simulink model "ASM2d_Influentmodel"  (Simulink 7.0)
settings: Solver=ode45  StartTime=0.0  StopTime=728.0  RelTol=1e-6
values from neighbouring files (symbols this model uses):
  aHpercent = 75    [ASM2d_Influent_init.m]    (also in ASM3_Influent_init.m)
  CODpart_gperPEperd = 115.08    [ASM2d_Influent_init.m]    (also in ASM3_Influent_init.m)
  CODpart_HH_max = 20*CODpart_gperPEperd*PE    (= 184128)    [ASM2d_Influent_init.m]    (also in ASM3_Influent_init.m)
  CODpart_HH_min = 0.1    [ASM2d_Influent_init.m]    (also in ASM3_Influent_init.m)
  CODpart_HH_ns = 35000    [ASM2d_Influent_init.m]    (also in ASM3_Influent_init.m)
  CODpart_HH_nv = factor1*CODpart_gperPEperd*PE    (= 18412.8)    [ASM2d_Influent_init.m]    (also in ASM3_Influent_init.m)
  CODpart_HH_st = 1/24    (= 0.0416666666667)    [ASM2d_Influent_init.m]    (also in ASM3_Influent_init.m)
  CODpart_Ind_kgperd = 2301.80    (= 2301.8)    [ASM2d_Influent_init.m]    (also in ASM3_Influent_init.m)
  CODpart_Ind_max = 20*CODpart_Ind_kgperd    (= 46036)    [ASM2d_Influent_init.m]    (also in ASM3_Influent_init.m)
  CODpart_Ind_min = 0.1    [ASM2d_Influent_init.m]    (also in ASM3_Influent_init.m)
  CODpart_Ind_ns = 21000    [ASM2d_Influent_init.m]    (also in ASM3_Influent_init.m)
  CODpart_Ind_nv = factor2*CODpart_Ind_kgperd    (= 4603.6)    [ASM2d_Influent_init.m]    (also in ASM3_Influent_init.m)
  CODpart_Ind_st = 1/24    (= 0.0416666666667)    [ASM2d_Influent_init.m]    (also in ASM3_Influent_init.m)
  CODsol_gperPEperd = 19.31    [ASM2d_Influent_init.m]    (also in ASM3_Influent_init.m)
  CODsol_HH_max = 20*CODsol_gperPEperd*PE    (= 30896)    [ASM2d_Influent_init.m]    (also in ASM3_Influent_init.m)
  CODsol_HH_min = 0.1    [ASM2d_Influent_init.m]    (also in ASM3_Influent_init.m)
  CODsol_HH_ns = 25000    [ASM2d_Influent_init.m]    (also in ASM3_Influent_init.m)
  CODsol_HH_nv = factor1*2*CODsol_gperPEperd*PE    (= 6179.2)    [ASM2d_Influent_init.m]    (also in ASM3_Influent_init.m)
  CODsol_HH_st = 1/24    (= 0.0416666666667)    [ASM2d_Influent_init.m]    (also in ASM3_Influent_init.m)
  CODsol_Ind_kgperd = 386.24    [ASM2d_Influent_init.m]    (also in ASM3_Influent_init.m)
  CODsol_Ind_max = 20*CODsol_Ind_kgperd    (= 7724.8)    [ASM2d_Influent_init.m]    (also in ASM3_Influent_init.m)
  CODsol_Ind_min = 0.1    [ASM2d_Influent_init.m]    (also in ASM3_Influent_init.m)
  CODsol_Ind_ns = 11000    [ASM2d_Influent_init.m]    (also in ASM3_Influent_init.m)
  CODsol_Ind_nv = factor2*CODsol_Ind_kgperd    (= 772.48)    [ASM2d_Influent_init.m]    (also in ASM3_Influent_init.m)
  CODsol_Ind_st = 1/24    (= 0.0416666666667)    [ASM2d_Influent_init.m]    (also in ASM3_Influent_init.m)
  FFfraction = 0.25    [ASM2d_Influent_init.m]    (also in ASM3_Influent_init.m)
  HHnoiseswitch = 1    [ASM2d_Influent_init.m]    (also in ASM3_Influent_init.m)
  HHpolnoiseswitch = 1    [ASM2d_Influent_init.m]    (also in ASM3_Influent_init.m)
  HHpopswitch = 100    [ASM2d_Influent_init.m]    (also in ASM3_Influent_init.m)
  Indnoiseswitch = 1    [ASM2d_Influent_init.m]    (also in ASM3_Influent_init.m)
  Indpolnoiseswitch = 1    [ASM2d_Influent_init.m]    (also in ASM3_Influent_init.m)
  Indpopswitch = 100    [ASM2d_Influent_init.m]    (also in ASM3_Influent_init.m)
  InfAmp = 1200    [ASM2d_Influent_init.m]    (also in ASM3_Influent_init.m)
  InfBias = 7100    [ASM2d_Influent_init.m]    (also in ASM3_Influent_init.m)
  Infcst = 7100    [ASM2d_Influent_init.m]    (also in ASM3_Influent_init.m)
  InfFreq = 2*pi/364    (= 0.0172614980966)    [ASM2d_Influent_init.m]    (also in ASM3_Influent_init.m)
  InfPhase = -pi*15/24    (= -1.96349540849)    [ASM2d_Influent_init.m]    (also in ASM3_Influent_init.m)
  iSS_XB = 0.90    (= 0.9)    [ASM2d_Influent_init.m]
  iSS_XI = 0.75    [ASM2d_Influent_init.m]
  iSS_XMe = 1.00    (= 1)    [ASM2d_Influent_init.m]
  iSS_XPHA = 0.60    (= 0.6)    [ASM2d_Influent_init.m]
  iSS_XPP = 3.23    [ASM2d_Influent_init.m]
  iSS_XS = 0.75    [ASM2d_Influent_init.m]
  LLrain = 3.5    [ASM2d_Influent_init.m]    (also in ASM3_Influent_init.m)
  PE = 80    [ASM2d_Influent_init.m]    (also in ASM3_Influent_init.m)
  PO4_gperPEperd = (6.89*0.85)/4    (= 1.464125)    [ASM2d_Influent_init.m]
  PO4_HH_max = 20*PO4_gperPEperd*PE    (= 2342.6)    [ASM2d_Influent_init.m]
  PO4_HH_min = 0.1    [ASM2d_Influent_init.m]
  PO4_HH_ns = 55000    [ASM2d_Influent_init.m]
  PO4_HH_nv = factor1*2*PO4_gperPEperd*PE    (= 468.52)    [ASM2d_Influent_init.m]
  PO4_HH_st = 1/24    (= 0.0416666666667)    [ASM2d_Influent_init.m]
  PO4_Ind_kgperd = (61.25*0.85)/4    (= 13.015625)    [ASM2d_Influent_init.m]
  PO4_Ind_max = 20*PO4_Ind_kgperd    (= 260.3125)    [ASM2d_Influent_init.m]
  PO4_Ind_min = 0.1    [ASM2d_Influent_init.m]
  PO4_Ind_ns = 41000    [ASM2d_Influent_init.m]
  PO4_Ind_nv = factor2*PO4_Ind_kgperd    (= 26.03125)    [ASM2d_Influent_init.m]
  PO4_Ind_st = 1/24    (= 0.0416666666667)    [ASM2d_Influent_init.m]
  polnoiseswitch = 1    [ASM2d_Influent_init.m]    (also in ASM3_Influent_init.m)
  Q_HH_ns = 3857    [ASM2d_Influent_init.m]    (also in ASM3_Influent_init.m)
  Q_HH_nv = 4000    [ASM2d_Influent_init.m]    (also in ASM3_Influent_init.m)
  Q_HH_st = 1/24    (= 0.0416666666667)    [ASM2d_Influent_init.m]    (also in ASM3_Influent_init.m)
  Q_Ind_ns = 2000    [ASM2d_Influent_init.m]    (also in ASM3_Influent_init.m)
  Q_Ind_nv = 15000    [ASM2d_Influent_init.m]    (also in ASM3_Influent_init.m)
  Q_Ind_st = 1/24    (= 0.0416666666667)    [ASM2d_Influent_init.m]    (also in ASM3_Influent_init.m)
  Q_SCI_ns = 1000    [ASM2d_Influent_init.m]    (also in ASM3_Influent_init.m)
  Q_SCI_nv = 0.1*InfBias    (= 710)    [ASM2d_Influent_init.m]    (also in ASM3_Influent_init.m)
  Q_SCI_st = 1    [ASM2d_Influent_init.m]    (also in ASM3_Influent_init.m)
  QHHsatmax = QperPE*50    (= 7500)    [ASM2d_Influent_init.m]    (also in ASM3_Influent_init.m)
  QHHsatmin = 0.001    [ASM2d_Influent_init.m]    (also in ASM3_Influent_init.m)
  QInd_weekday = 2500    [ASM2d_Influent_init.m]    (also in ASM3_Influent_init.m)
  QIndsatmax = QInd_weekday*10    (= 25000)    [ASM2d_Influent_init.m]    (also in ASM3_Influent_init.m)
  QIndsatmin = 0.001    [ASM2d_Influent_init.m]    (also in ASM3_Influent_init.m)
  Qpermm = 1500    [ASM2d_Influent_init.m]    (also in ASM3_Influent_init.m)
  QperPE = 150    [ASM2d_Influent_init.m]    (also in ASM3_Influent_init.m)
  QSCIsatmax = 2*(InfBias+InfAmp)    (= 16600)    [ASM2d_Influent_init.m]    (also in ASM3_Influent_init.m)
  QSCIsatmin = 0.0    (= 0)    [ASM2d_Influent_init.m]    (also in ASM3_Influent_init.m)
  rain_nm = 1    [ASM2d_Influent_init.m]    (also in ASM3_Influent_init.m)
  rain_ns = 3000    [ASM2d_Influent_init.m]    (also in ASM3_Influent_init.m)
  rain_nv = 400    [ASM2d_Influent_init.m]    (also in ASM3_Influent_init.m)
  rain_st = 1/24    (= 0.0416666666667)    [ASM2d_Influent_init.m]    (also in ASM3_Influent_init.m)
  rainmax = 1000    [ASM2d_Influent_init.m]    (also in ASM3_Influent_init.m)
  rainmin = 0    [ASM2d_Influent_init.m]    (also in ASM3_Influent_init.m)
  rainpopswitch = 100    [ASM2d_Influent_init.m]    (also in ASM3_Influent_init.m)
  SA_max = 100*Sa_in    (= 2780)    [ASM2d_Influent_init.m]
  SA_min = 0.1    [ASM2d_Influent_init.m]
  SA_ns = 03122    (= 3122)    [ASM2d_Influent_init.m]
  SA_nv = factor3*(Sa_in)    (= 55.6)    [ASM2d_Influent_init.m]
  SA_st = 1/24    (= 0.0416666666667)    [ASM2d_Influent_init.m]
  SCInoiseswitch = 0    [ASM2d_Influent_init.m]    (also in ASM3_Influent_init.m)
  SCIpopswitch = 100    [ASM2d_Influent_init.m]    (also in ASM3_Influent_init.m)
  SF_max = 100*Sf_in    (= 4170)    [ASM2d_Influent_init.m]
  SF_min = 0.1    [ASM2d_Influent_init.m]
  SF_ns = 23122    [ASM2d_Influent_init.m]
  SF_nv = factor3*(Sf_in)    (= 83.4)    [ASM2d_Influent_init.m]
  SF_st = 1/24    (= 0.0416666666667)    [ASM2d_Influent_init.m]
  SI_max = 100*Si_in    (= 3000)    [ASM2d_Influent_init.m]    (also in ASM3_Influent_init.m)
  SI_min = 0.1    [ASM2d_Influent_init.m]    (also in ASM3_Influent_init.m)
  SI_ns = 13122    [ASM2d_Influent_init.m]    (also in ASM3_Influent_init.m)
  SI_nv = factor3*(Si_in)    (= 60)    [ASM2d_Influent_init.m]    (also in ASM3_Influent_init.m)
  SI_st = 1/24    (= 0.0416666666667)    [ASM2d_Influent_init.m]    (also in ASM3_Influent_init.m)
  SNH_gperPEperd = 6.89*0.85    (= 5.8565)    [ASM2d_Influent_init.m]    (also in ASM3_Influent_init.m)
  SNH_HH_max = 20*SNH_gperPEperd*PE    (= 9370.4)    [ASM2d_Influent_init.m]    (also in ASM3_Influent_init.m)
  SNH_HH_min = 0.1    [ASM2d_Influent_init.m]    (also in ASM3_Influent_init.m)
  SNH_HH_ns = 45000    [ASM2d_Influent_init.m]    (also in ASM3_Influent_init.m)
  SNH_HH_nv = factor1*2*SNH_gperPEperd*PE    (= 1874.08)    [ASM2d_Influent_init.m]    (also in ASM3_Influent_init.m)
  SNH_HH_st = 1/24    (= 0.0416666666667)    [ASM2d_Influent_init.m]    (also in ASM3_Influent_init.m)
  SNH_Ind_kgperd = 61.25*0.85    (= 52.0625)    [ASM2d_Influent_init.m]    (also in ASM3_Influent_init.m)
  SNH_Ind_max = 20*SNH_Ind_kgperd    (= 1041.25)    [ASM2d_Influent_init.m]    (also in ASM3_Influent_init.m)
  SNH_Ind_min = 0.1    [ASM2d_Influent_init.m]    (also in ASM3_Influent_init.m)
  SNH_Ind_ns = 31000    [ASM2d_Influent_init.m]    (also in ASM3_Influent_init.m)
  SNH_Ind_nv = factor2*SNH_Ind_kgperd    (= 104.125)    [ASM2d_Influent_init.m]    (also in ASM3_Influent_init.m)
  SNH_Ind_st = 1/24    (= 0.0416666666667)    [ASM2d_Influent_init.m]    (also in ASM3_Influent_init.m)
  SNH_max = 100*Snh_in    (= 3156)    [ASM2d_Influent_init.m]    (also in ASM3_Influent_init.m)
  SNH_min = 0.1    [ASM2d_Influent_init.m]    (also in ASM3_Influent_init.m)
  SNH_ns = 63122    [ASM2d_Influent_init.m]    (also in ASM3_Influent_init.m)
  SNH_nv = factor3*(Snh_in)    (= 63.12)    [ASM2d_Influent_init.m]    (also in ASM3_Influent_init.m)
  SNH_st = 1/24    (= 0.0416666666667)    [ASM2d_Influent_init.m]    (also in ASM3_Influent_init.m)
  SPO4_ns = 73122    [ASM2d_Influent_init.m]
  SPO4_nv = factor3*(Spo4_in)    (= 18.02)    [ASM2d_Influent_init.m]
  SPO4_st = 1/24    (= 0.0416666666667)    [ASM2d_Influent_init.m]
  ... (+24 more)
libraries: simulink x5
(part 1 of 2)
Description:
  | BSM2 influent model, version 15 March 2005
settings Model: Creator=Krist V. Gernaey  LastModifiedBy=xavier  ExtModeAutoUpdateStatusClock=off
settings DataIOCC: LimitDataPoints=off  SignalLoggingName=sigsOut  OutputOption=SpecifiedOutputTimes  OutputTimes=[119:1.0/96.0:728.0]
settings DebuggingCC: SaveWithParameterizedLinksMsg=none  SignalResolutionControl=TryResolveAllWithWarning  SolverPrmCheckMsg=none  MultiTaskDSMMsg=warning  MultiTaskCondExecSysMsg=none  StrictBusMsg=None
settings HardwareCC: TargetEndianess=LittleEndian  TargetHWDeviceType=MATLAB Host  ProdEqTarget=off
settings RTWCC: IncludeERTFirstTime=on

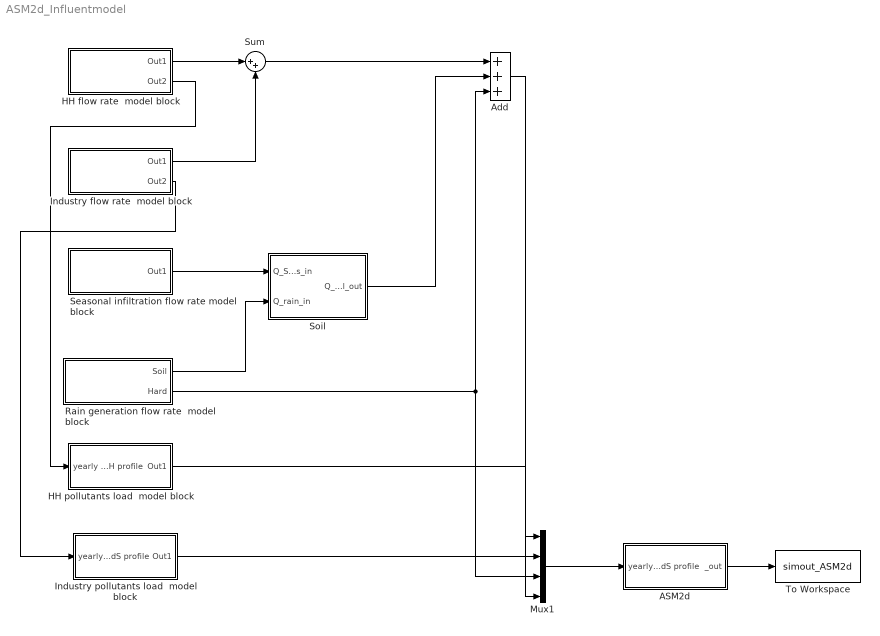
== system ASM2d_Influentmodel ==
  ASM2d : Subsystem
  Add : Sum  Inputs=+++  OutDataType=sfix(16)  OutScaling=2^-10
  HH flow rate  model block : Subsystem
  "HH pollutants load  model block " : Subsystem
  Industry flow rate  model block : Subsystem
  "Industry pollutants load  model block " : Subsystem
  Mux1 : Mux
  Rain generation flow rate  model block : Subsystem
  Seasonal infiltration flow rate model block : Subsystem
  Soil : Subsystem
  Sum : Sum  Inputs=|++  OutDataType=sfix(16)  OutScaling=2^0  SaturateOnIntegerOverflow=on
  To Workspace : ToWorkspace  VariableName=simout_ASM2d  SampleTime=-1  SaveFormat=Array
  wires:
  Add/1 -> Mux1/4
  Rain generation flow rate  model block/2(Hard) -> Mux1/3, Add/3
  Soil/1(Q_Soil_out) -> Add/2
  Sum/1 -> Add/1
  HH flow rate  model block/1(Out1) -> Sum/1
  Rain generation flow rate  model block/1(Soil) -> Soil/2(Q_rain_in)
  Seasonal infiltration flow rate model block/1(Out1) -> Soil/1(Q_Seas_in)
  Industry flow rate  model block/1(Out1) -> Sum/2
  HH flow rate  model block/2(Out2) -> "HH pollutants load  model block "/1(yearly HH profile)
  Industry flow rate  model block/2(Out2) -> "Industry pollutants load  model block "/1(yearly_indS profile)
  "HH pollutants load  model block "/1(Out1) -> Mux1/1
  "Industry pollutants load  model block "/1(Out1) -> Mux1/2
  Mux1/1 -> ASM2d/1(yearly_indS profile)
  ASM2d/1(_out) -> To Workspace/1

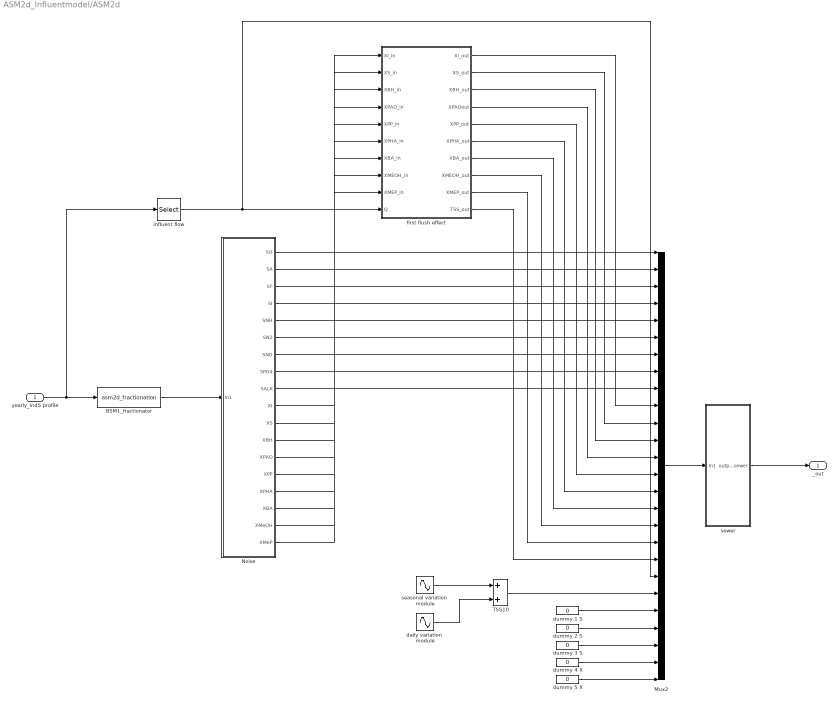
== system ASM2d_Influentmodel/ASM2d ==
  yearly_indS profile : Inport  OutDataType=sfix(16)  OutScaling=2^0
  BSM1_fractionator : S-Function  FunctionName=asm2d_fractionation  Parameters=ASM2d_PARS, ASM2d_FRACTIONS
  Mux2 : Mux  Inputs=26
  Noise : Subsystem
  TSS10 : Sum  OutDataType=sfix(16)  OutScaling=2^-10
  daily variation  module : Sin  Amplitude=TdAmp  Bias=TdBias  Frequency=TdFreq  Phase=TdPhase  SampleTime=0
  dummy 1 S : Constant  Value=0  OutDataType=sfix(16)  OutScaling=2^0
  dummy 2 S : Constant  Value=0  OutDataType=sfix(16)  OutScaling=2^0
  dummy 3 S : Constant  Value=0  OutDataType=sfix(16)  OutScaling=2^0
  dummy 4 X : Constant  Value=0  OutDataType=sfix(16)  OutScaling=2^0
  dummy 5 X : Constant  Value=0  OutDataType=sfix(16)  OutScaling=2^0
  first flush effect : Subsystem
  influent flow : Selector  InputPortWidth=12  IndexOptions=Index vector (dialog)  Indices=[12]  OutputSizes=1
  seasonal variation  module : Sin  Amplitude=TAmp  Bias=TBias  Frequency=TFreq  Phase=TPhase  SampleTime=0
  sewer : Subsystem
  _out : Outport  OutDataType=sfix(16)  OutScaling=2^0
  wires:
  yearly_indS profile/1 -> BSM1_fractionator/1, influent flow/1
  Noise/10(XI) -> first flush effect/1(XI_in)
  Noise/11(XS) -> first flush effect/2(XS_in)
  Noise/12(XBH) -> first flush effect/3(XBH_in)
  Noise/13(XPAO) -> first flush effect/4(XPAO_in)
  Noise/14(XPP) -> first flush effect/5(XPP_in)
  Noise/15(XPHA) -> first flush effect/6(XPHA_in)
  Noise/16(XBA) -> first flush effect/7(XBA_in)
  Noise/17(XMeOH) -> first flush effect/8(XMEOH_in)
  Noise/18(XMeP) -> first flush effect/9(XMEP_in)
  BSM1_fractionator/1 -> Noise/1(In1)
  influent flow/1 -> first flush effect/10(Q), Mux2/20
  Noise/1(SO) -> Mux2/1
  Noise/2(SA) -> Mux2/2
  Noise/3(SF) -> Mux2/3
  Noise/4(SI) -> Mux2/4
  Noise/5(SNH) -> Mux2/5
  Noise/6(SN2) -> Mux2/6
  Noise/7(SNO) -> Mux2/7
  Noise/8(SPO4) -> Mux2/8
  Noise/9(SALK) -> Mux2/9
  first flush effect/1(XI_out) -> Mux2/10
  first flush effect/2(XS_out) -> Mux2/11
  first flush effect/3(XBH_out) -> Mux2/12
  first flush effect/4(XPAOout) -> Mux2/13
  first flush effect/5(XPP_out) -> Mux2/14
  first flush effect/6(XPHA_out) -> Mux2/15
  first flush effect/7(XBA_out) -> Mux2/16
  first flush effect/8(XMEOH_out) -> Mux2/17
  first flush effect/9(XMEP_out) -> Mux2/18
  first flush effect/10(TSS_out) -> Mux2/19
  dummy 5 X/1 -> Mux2/26
  dummy 4 X/1 -> Mux2/25
  dummy 3 S/1 -> Mux2/24
  dummy 2 S/1 -> Mux2/23
  dummy 1 S/1 -> Mux2/22
  Mux2/1 -> sewer/1(In1)
  sewer/1(output sewer) -> _out/1
  TSS10/1 -> Mux2/21
  seasonal variation  module/1 -> TSS10/1
  daily variation  module/1 -> TSS10/2

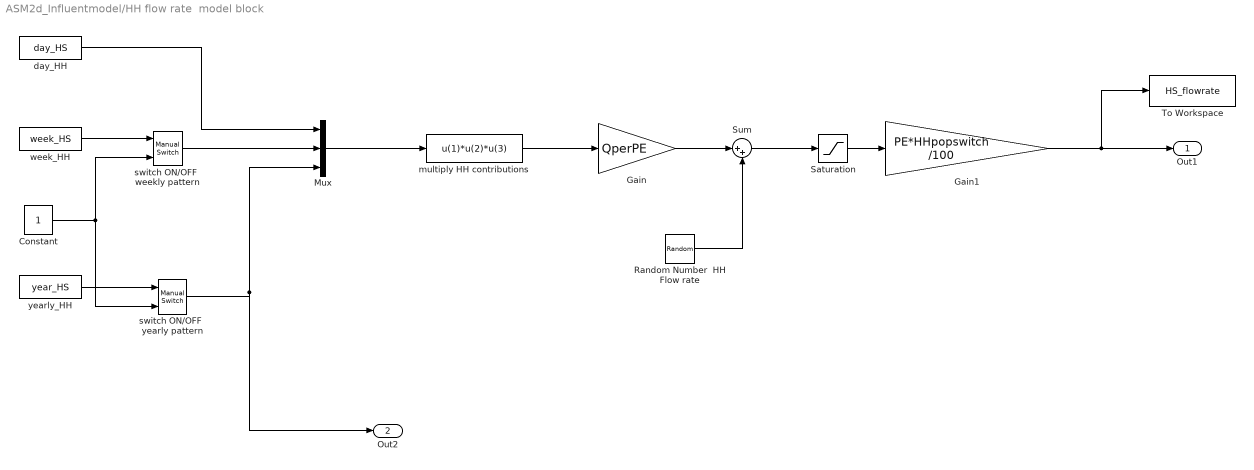
== system ASM2d_Influentmodel/HH flow rate  model block ==
  Constant : Constant  OutDataType=sfix(16)  OutScaling=2^0
  Gain : Gain  Gain=QperPE  ParameterDataType=sfix(16)  ParameterScaling=2^0  OutDataType=sfix(16)  OutScaling=2^0
  Gain1 : Gain  Gain=PE*HHpopswitch /100  ParameterDataType=sfix(16)  ParameterScaling=2^0  OutDataType=sfix(16)  OutScaling=2^0
  Mux : Mux  Inputs=3
  Random Number  HH Flow rate : RandomNumber  Variance=Q_HH_nv*HHnoiseswitch  Seed=Q_HH_ns  SampleTime=Q_HH_st
  Saturation : Saturate  UpperLimit=QHHsatmax  LowerLimit=QHHsatmin  OutDataType=sfix(16)  OutScaling=2^0
  Sum : Sum  Inputs=|++  OutDataType=sfix(16)  OutScaling=2^0
  To Workspace : ToWorkspace  VariableName=HS_flowrate  SampleTime=-1  SaveFormat=Array
  day_HH : FromWorkspace  VariableName=day_HS  SampleTime=1/24  Interpolate=off  OutputAfterFinalValue=Cyclic repetition
  multiply HH contributions : Fcn  Expr=u(1)*u(2)*u(3)
  switch ON/OFF  weekly pattern : simulink/Signal Routing/Manual Switch  SystemSampleTime=-1  sw=1  action=0  varsize=off
  switch ON/OFF  yearly pattern : simulink/Signal Routing/Manual Switch  SystemSampleTime=-1  sw=1  action=0  varsize=off
  week_HH : FromWorkspace  VariableName=week_HS  SampleTime=1  Interpolate=off  OutputAfterFinalValue=Cyclic repetition
  yearly_HH : FromWorkspace  VariableName=year_HS  SampleTime=1  Interpolate=off  OutputAfterFinalValue=Cyclic repetition
  Out1 : Outport  OutDataType=sfix(16)  OutScaling=2^0
  Out2 : Outport  Port=2  OutDataType=sfix(16)  OutScaling=2^0
  wires:
  multiply HH contributions/1 -> Gain/1
  Gain/1 -> Sum/1
  Sum/1 -> Saturation/1
  Saturation/1 -> Gain1/1
  Gain1/1 -> Out1/1, To Workspace/1
  Random Number  HH Flow rate/1 -> Sum/2
  week_HH/1 -> switch ON/OFF  weekly pattern/1
  yearly_HH/1 -> switch ON/OFF  yearly pattern/1
  day_HH/1 -> Mux/1
  switch ON/OFF  weekly pattern/1 -> Mux/2
  switch ON/OFF  yearly pattern/1 -> Mux/3, Out2/1
  Constant/1 -> switch ON/OFF  weekly pattern/2, switch ON/OFF  yearly pattern/2
  Mux/1 -> multiply HH contributions/1

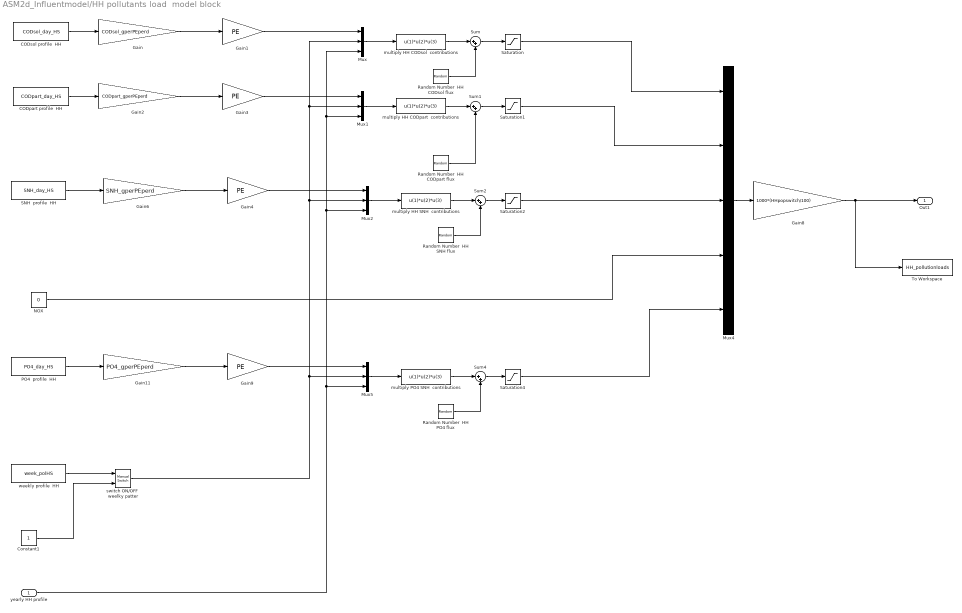
== system ASM2d_Influentmodel/HH pollutants load  model block  ==
  yearly HH profile : Inport  OutDataType=sfix(16)  OutScaling=2^0
  CODpart profile  HH : FromWorkspace  VariableName=CODpart_day_HS  SampleTime=1/24  Interpolate=off  OutputAfterFinalValue=Cyclic repetition
  CODsol profile  HH : FromWorkspace  VariableName=CODsol_day_HS  SampleTime=1/24  Interpolate=off  OutputAfterFinalValue=Cyclic repetition
  Constant1 : Constant  OutDataType=sfix(16)  OutScaling=2^0
  Gain : Gain  Gain=CODsol_gperPEperd  ParameterDataType=sfix(16)  ParameterScaling=2^0  OutDataType=sfix(16)  OutScaling=2^0
  Gain{1,3..4,9} (4 alike) : Gain  Gain=PE  ParameterDataType=sfix(16)  ParameterScaling=2^0  OutDataType=sfix(16)  OutScaling=2^0
  Gain11 : Gain  Gain=PO4_gperPEperd  ParameterDataType=sfix(16)  ParameterScaling=2^0  OutDataType=sfix(16)  OutScaling=2^0
  Gain2 : Gain  Gain=CODpart_gperPEperd  ParameterDataType=sfix(16)  ParameterScaling=2^0  OutDataType=sfix(16)  OutScaling=2^0
  Gain6 : Gain  Gain=SNH_gperPEperd  ParameterDataType=sfix(16)  ParameterScaling=2^0  OutDataType=sfix(16)  OutScaling=2^0
  Gain8 : Gain  Gain=1000*(HHpopswitch/100)  ParameterDataType=sfix(16)  ParameterScaling=2^0  OutDataType=sfix(16)  OutScaling=2^0
  Mux{,1..2,5} (4 alike) : Mux  Inputs=3
  Mux4 : Mux  Inputs=5
  NOX : Constant  Value=0  OutDataType=sfix(16)  OutScaling=2^0
  PO4  profile  HH : FromWorkspace  VariableName=PO4_day_HS  SampleTime=1/24  Interpolate=off  OutputAfterFinalValue=Cyclic repetition
  Random Number  HH CODpart flux : RandomNumber  Variance=CODpart_HH_nv*HHpolnoiseswitch  Seed=CODpart_HH_ns  SampleTime=CODpart_HH_st
  Random Number  HH CODsol flux : RandomNumber  Variance=CODsol_HH_nv*HHpolnoiseswitch  Seed=CODsol_HH_ns  SampleTime=CODsol_HH_st
  Random Number  HH PO4 flux : RandomNumber  Variance=PO4_HH_nv*HHpolnoiseswitch  Seed=PO4_HH_ns  SampleTime=PO4_HH_st
  Random Number  HH SNH flux : RandomNumber  Variance=SNH_HH_nv*HHpolnoiseswitch  Seed=SNH_HH_ns  SampleTime=SNH_HH_st
  SNH  profile  HH : FromWorkspace  VariableName=SNH_day_HS  SampleTime=1/24  Interpolate=off  OutputAfterFinalValue=Cyclic repetition
  Saturation : Saturate  UpperLimit=CODsol_HH_max  LowerLimit=CODsol_HH_min  OutDataType=sfix(16)  OutScaling=2^0
  Saturation1 : Saturate  UpperLimit=CODpart_HH_max  LowerLimit=CODpart_HH_min  OutDataType=sfix(16)  OutScaling=2^0
  Saturation2 : Saturate  UpperLimit=SNH_HH_max  LowerLimit=SNH_HH_min  OutDataType=sfix(16)  OutScaling=2^0
  Saturation4 : Saturate  UpperLimit=PO4_HH_max  LowerLimit=PO4_HH_min  OutDataType=sfix(16)  OutScaling=2^0
  Sum{,1..2,4} (4 alike) : Sum  Inputs=|++  OutDataType=sfix(16)  OutScaling=2^0
  To Workspace : ToWorkspace  VariableName=HH_pollutionloads  SampleTime=-1  SaveFormat=Array
  multiply HH CODpart  contributions : Fcn  Expr=u(1)*u(2)*u(3)
  multiply HH CODsol  contributions : Fcn  Expr=u(1)*u(2)*u(3)
  multiply HH SNH  contributions : Fcn  Expr=u(1)*u(2)*u(3)
  multiply PO4 SNH  contributions : Fcn  Expr=u(1)*u(2)*u(3)
  switch ON/OFF  weelky patter : simulink/Signal Routing/Manual Switch  SystemSampleTime=-1  sw=1  action=0  varsize=off
  weekly profile  HH : FromWorkspace  VariableName=week_polHS  SampleTime=1  Interpolate=off  OutputAfterFinalValue=Cyclic repetition
  Out1 : Outport  OutDataType=sfix(16)  OutScaling=2^0
  wires:
  Random Number  HH CODsol flux/1 -> Sum/2
  CODsol profile  HH/1 -> Gain/1
  Gain/1 -> Gain1/1
  Mux/1 -> multiply HH CODsol  contributions/1
  multiply HH CODsol  contributions/1 -> Sum/1
  Sum/1 -> Saturation/1
  Gain1/1 -> Mux/1
  Random Number  HH CODpart flux/1 -> Sum1/2
  CODpart profile  HH/1 -> Gain2/1
  Gain2/1 -> Gain3/1
  Mux1/1 -> multiply HH CODpart  contributions/1
  multiply HH CODpart  contributions/1 -> Sum1/1
  Sum1/1 -> Saturation1/1
  Gain3/1 -> Mux1/1
  Random Number  HH SNH flux/1 -> Sum2/2
  SNH  profile  HH/1 -> Gain6/1
  Gain6/1 -> Gain4/1
  Mux2/1 -> multiply HH SNH  contributions/1
  multiply HH SNH  contributions/1 -> Sum2/1
  Sum2/1 -> Saturation2/1
  Gain4/1 -> Mux2/1
  Mux4/1 -> Gain8/1
  Constant1/1 -> switch ON/OFF  weelky patter/2
  weekly profile  HH/1 -> switch ON/OFF  weelky patter/1
  Random Number  HH PO4 flux/1 -> Sum4/2
  PO4  profile  HH/1 -> Gain11/1
  Gain11/1 -> Gain9/1
  Mux5/1 -> multiply PO4 SNH  contributions/1
  multiply PO4 SNH  contributions/1 -> Sum4/1
  Sum4/1 -> Saturation4/1
  Gain9/1 -> Mux5/1
  Saturation/1 -> Mux4/1
  Saturation1/1 -> Mux4/2
  Saturation2/1 -> Mux4/3
  Saturation4/1 -> Mux4/5
  switch ON/OFF  weelky patter/1 -> Mux5/2, Mux2/2, Mux/2, Mux1/2
  yearly HH profile/1 -> Mux5/3, Mux2/3, Mux/3, Mux1/3
  Gain8/1 -> Out1/1, To Workspace/1
  NOX/1 -> Mux4/4

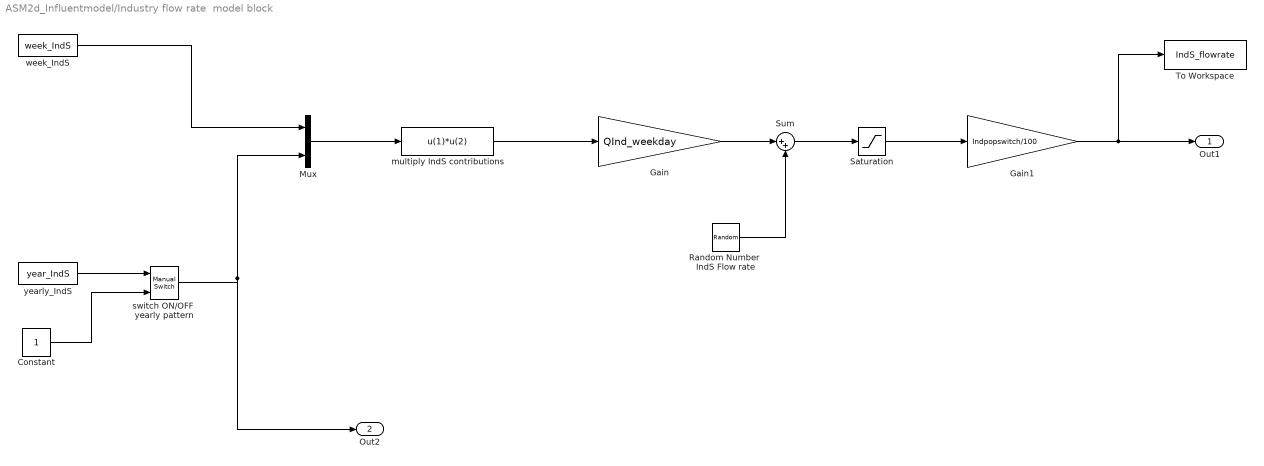
== system ASM2d_Influentmodel/Industry flow rate  model block ==
  Constant : Constant  OutDataType=sfix(16)  OutScaling=2^0
  Gain : Gain  Gain=QInd_weekday  ParameterDataType=sfix(16)  ParameterScaling=2^0  OutDataType=sfix(16)  OutScaling=2^0
  Gain1 : Gain  Gain=Indpopswitch/100  ParameterDataType=sfix(16)  ParameterScaling=2^0  OutDataType=sfix(16)  OutScaling=2^0
  Mux : Mux  Inputs=2
  Random Number  IndS Flow rate : RandomNumber  Variance=Q_Ind_nv*Indnoiseswitch  Seed=Q_Ind_ns  SampleTime=Q_Ind_st
  Saturation : Saturate  UpperLimit=QIndsatmax  LowerLimit=QIndsatmin  OutDataType=sfix(16)  OutScaling=2^0
  Sum : Sum  Inputs=|++  OutDataType=sfix(16)  OutScaling=2^0
  To Workspace : ToWorkspace  VariableName=IndS_flowrate  SampleTime=-1  SaveFormat=Array
  multiply IndS contributions : Fcn  Expr=u(1)*u(2)
  switch ON/OFF  yearly pattern : simulink/Signal Routing/Manual Switch  SystemSampleTime=-1  sw=1  action=0  varsize=off
  week_IndS : FromWorkspace  VariableName=week_IndS  SampleTime=1/6  Interpolate=off  OutputAfterFinalValue=Cyclic repetition
  yearly_IndS : FromWorkspace  VariableName=year_IndS  SampleTime=1  Interpolate=off  OutputAfterFinalValue=Cyclic repetition
  Out1 : Outport  OutDataType=sfix(16)  OutScaling=2^0
  Out2 : Outport  Port=2  OutDataType=sfix(16)  OutScaling=2^0
  wires:
  multiply IndS contributions/1 -> Gain/1
  Gain/1 -> Sum/1
  Sum/1 -> Saturation/1
  Saturation/1 -> Gain1/1
  Gain1/1 -> Out1/1, To Workspace/1
  Random Number  IndS Flow rate/1 -> Sum/2
  yearly_IndS/1 -> switch ON/OFF  yearly pattern/1
  week_IndS/1 -> Mux/1
  switch ON/OFF  yearly pattern/1 -> Mux/2, Out2/1
  Constant/1 -> switch ON/OFF  yearly pattern/2
  Mux/1 -> multiply IndS contributions/1

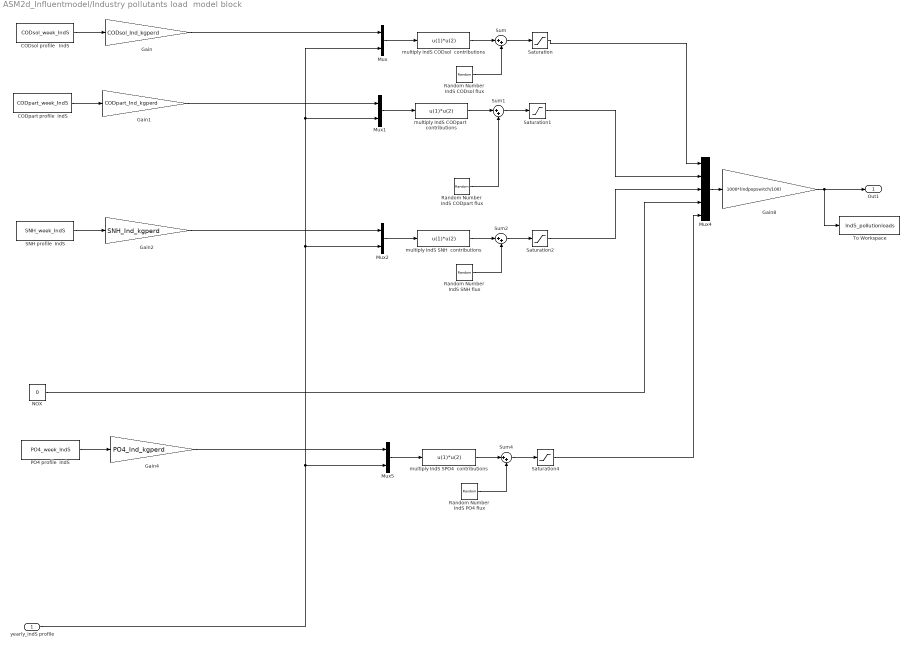
== system ASM2d_Influentmodel/Industry pollutants load  model block  ==
  yearly_indS profile : Inport  OutDataType=sfix(16)  OutScaling=2^0
  CODpart profile  IndS : FromWorkspace  VariableName=CODpart_week_IndS  SampleTime=1/6  Interpolate=off  OutputAfterFinalValue=Cyclic repetition
  CODsol profile   IndS : FromWorkspace  VariableName=CODsol_week_IndS  SampleTime=1/6  Interpolate=off  OutputAfterFinalValue=Cyclic repetition
  Gain : Gain  Gain=CODsol_Ind_kgperd  ParameterDataType=sfix(16)  ParameterScaling=2^0  OutDataType=sfix(16)  OutScaling=2^0
  Gain1 : Gain  Gain=CODpart_Ind_kgperd  ParameterDataType=sfix(16)  ParameterScaling=2^0  OutDataType=sfix(16)  OutScaling=2^0
  Gain2 : Gain  Gain=SNH_Ind_kgperd  ParameterDataType=sfix(16)  ParameterScaling=2^0  OutDataType=sfix(16)  OutScaling=2^0
  Gain4 : Gain  Gain=PO4_Ind_kgperd  ParameterDataType=sfix(16)  ParameterScaling=2^0  OutDataType=sfix(16)  OutScaling=2^0
  Gain8 : Gain  Gain=1000*(Indpopswitch/100)  ParameterDataType=sfix(16)  ParameterScaling=2^0  OutDataType=sfix(16)  OutScaling=2^0
  Mux{,1..2,5} (4 alike) : Mux  Inputs=2
  Mux4 : Mux  Inputs=5
  NOX : Constant  Value=0  OutDataType=sfix(16)  OutScaling=2^0
  PO4 profile  IndS : FromWorkspace  VariableName=PO4_week_IndS  SampleTime=1/6  Interpolate=off  OutputAfterFinalValue=Cyclic repetition
  Random Number  IndS CODpart flux : RandomNumber  Variance=CODpart_Ind_nv*Indpolnoiseswitch  Seed=CODpart_Ind_ns  SampleTime=CODpart_Ind_st
  Random Number  IndS CODsol flux : RandomNumber  Variance=CODsol_Ind_nv*Indpolnoiseswitch  Seed=CODsol_Ind_ns  SampleTime=CODsol_Ind_st
  Random Number  IndS PO4 flux : RandomNumber  Variance=PO4_Ind_nv*Indpolnoiseswitch  Seed=PO4_Ind_ns  SampleTime=PO4_Ind_st
  Random Number  IndS SNH flux : RandomNumber  Variance=SNH_Ind_nv*Indpolnoiseswitch  Seed=SNH_Ind_ns  SampleTime=SNH_Ind_st
  SNH profile  IndS : FromWorkspace  VariableName=SNH_week_IndS  SampleTime=1/6  Interpolate=off  OutputAfterFinalValue=Cyclic repetition
  Saturation : Saturate  UpperLimit=CODsol_Ind_max  LowerLimit=CODsol_Ind_min  OutDataType=sfix(16)  OutScaling=2^0
  Saturation1 : Saturate  UpperLimit=CODpart_Ind_max  LowerLimit=CODpart_Ind_min  OutDataType=sfix(16)  OutScaling=2^0
  Saturation2 : Saturate  UpperLimit=SNH_Ind_max  LowerLimit=SNH_Ind_min  OutDataType=sfix(16)  OutScaling=2^0
  Saturation4 : Saturate  UpperLimit=PO4_Ind_max  LowerLimit=PO4_Ind_min  OutDataType=sfix(16)  OutScaling=2^0
  Sum{,1..2,4} (4 alike) : Sum  Inputs=|++  OutDataType=sfix(16)  OutScaling=2^0
  To Workspace : ToWorkspace  VariableName=IndS_pollutionloads  SampleTime=-1  SaveFormat=Array
  multiply IndS CODpart  contributions : Fcn  Expr=u(1)*u(2)
  multiply IndS CODsol  contributions : Fcn  Expr=u(1)*u(2)
  multiply IndS SNH  contributions : Fcn  Expr=u(1)*u(2)
  multiply IndS SPO4  contributions : Fcn  Expr=u(1)*u(2)
  Out1 : Outport  OutDataType=sfix(16)  OutScaling=2^0
  wires:
  Random Number  IndS CODsol flux/1 -> Sum/2
  CODsol profile   IndS/1 -> Gain/1
  Mux/1 -> multiply IndS CODsol  contributions/1
  multiply IndS CODsol  contributions/1 -> Sum/1
  Sum/1 -> Saturation/1
  Mux4/1 -> Gain8/1
  Gain/1 -> Mux/1
  Random Number  IndS CODpart flux/1 -> Sum1/2
  CODpart profile  IndS/1 -> Gain1/1
  Mux1/1 -> multiply IndS CODpart  contributions/1
  multiply IndS CODpart  contributions/1 -> Sum1/1
  Sum1/1 -> Saturation1/1
  Gain1/1 -> Mux1/1
  Random Number  IndS SNH flux/1 -> Sum2/2
  SNH profile  IndS/1 -> Gain2/1
  Mux2/1 -> multiply IndS SNH  contributions/1
  multiply IndS SNH  contributions/1 -> Sum2/1
  Sum2/1 -> Saturation2/1
  Gain2/1 -> Mux2/1
  yearly_indS profile/1 -> Mux5/2, Mux2/2, Mux/2, Mux1/2
  Saturation/1 -> Mux4/1
  Saturation1/1 -> Mux4/2
  Saturation2/1 -> Mux4/3
  Random Number  IndS PO4 flux/1 -> Sum4/2
  PO4 profile  IndS/1 -> Gain4/1
  Mux5/1 -> multiply IndS SPO4  contributions/1
  multiply IndS SPO4  contributions/1 -> Sum4/1
  Sum4/1 -> Saturation4/1
  Gain4/1 -> Mux5/1
  Gain8/1 -> Out1/1, To Workspace/1
  NOX/1 -> Mux4/4
  Saturation4/1 -> Mux4/5

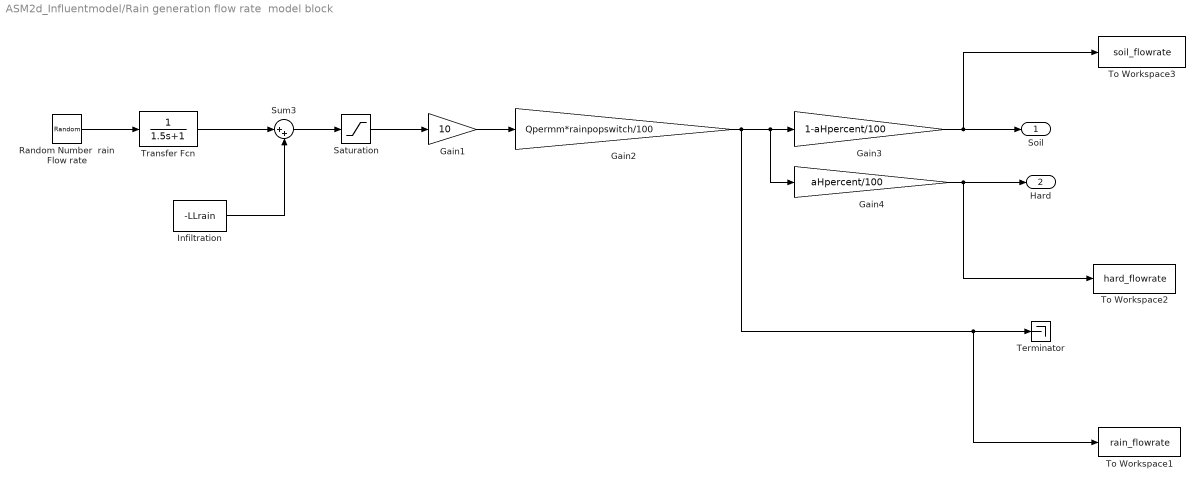
== system ASM2d_Influentmodel/Rain generation flow rate  model block ==
  Gain1 : Gain  Gain=10  ParameterDataType=sfix(16)  ParameterScaling=2^0  OutDataType=sfix(16)  OutScaling=2^0  SaturateOnIntegerOverflow=on
  Gain2 : Gain  Gain=Qpermm*rainpopswitch/100  ParameterDataType=sfix(16)  ParameterScaling=2^0  OutDataType=sfix(16)  OutScaling=2^0  SaturateOnIntegerOverflow=on
  Gain3 : Gain  Gain=1-aHpercent/100  ParameterDataType=sfix(16)  ParameterScaling=2^0  OutDataType=sfix(16)  OutScaling=2^0  SaturateOnIntegerOverflow=on
  Gain4 : Gain  Gain=aHpercent/100  ParameterDataType=sfix(16)  ParameterScaling=2^0  OutDataType=sfix(16)  OutScaling=2^0  SaturateOnIntegerOverflow=on
  Infiltration : Constant  Value=-LLrain  OutDataType=sfix(16)  OutScaling=2^0
  Random Number  rain Flow rate : RandomNumber  Mean=rain_nm  Variance=rain_nv  Seed=rain_ns  SampleTime=rain_st
  Saturation : Saturate  UpperLimit=rainmax  LowerLimit=rainmin
  Sum3 : Sum  Inputs=|++  OutDataType=sfix(16)  OutScaling=2^0  SaturateOnIntegerOverflow=on
  Terminator : Terminator
  To Workspace1 : ToWorkspace  VariableName=rain_flowrate  SampleTime=-1  SaveFormat=Array
  To Workspace2 : ToWorkspace  VariableName=hard_flowrate  SampleTime=-1  SaveFormat=Array
  To Workspace3 : ToWorkspace  VariableName=soil_flowrate  SampleTime=-1  SaveFormat=Array
  Transfer Fcn : TransferFcn  Denominator=[1.5 1]
  Soil : Outport
  Hard : Outport  Port=2
  wires:
  Random Number  rain Flow rate/1 -> Transfer Fcn/1
  Gain3/1 -> Soil/1, To Workspace3/1
  Gain4/1 -> Hard/1, To Workspace2/1
  Gain2/1 -> Gain4/1, Gain3/1, To Workspace1/1, Terminator/1
  Gain1/1 -> Gain2/1
  Saturation/1 -> Gain1/1
  Infiltration/1 -> Sum3/2
  Transfer Fcn/1 -> Sum3/1
  Sum3/1 -> Saturation/1

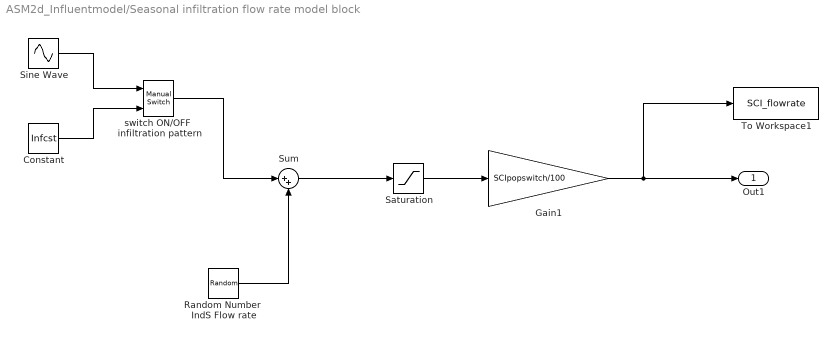
== system ASM2d_Influentmodel/Seasonal infiltration flow rate model block ==
  Constant : Constant  Value=Infcst  OutDataType=sfix(16)  OutScaling=2^0
  Gain1 : Gain  Gain=SCIpopswitch/100  ParameterDataType=sfix(16)  ParameterScaling=2^0  OutDataType=sfix(16)  OutScaling=2^0
  Random Number  IndS Flow rate : RandomNumber  Variance=Q_SCI_nv*SCInoiseswitch  Seed=Q_SCI_ns  SampleTime=Q_SCI_st
  Saturation : Saturate  UpperLimit=QSCIsatmax  LowerLimit=QSCIsatmin  OutDataType=sfix(16)  OutScaling=2^0
  Sine Wave : Sin  Amplitude=InfAmp  Bias=InfBias  Frequency=InfFreq  Phase=InfPhase  SampleTime=0
  Sum : Sum  Inputs=|++  OutDataType=sfix(16)  OutScaling=2^0
  To Workspace1 : ToWorkspace  VariableName=SCI_flowrate  SampleTime=-1  SaveFormat=Array
  switch ON/OFF  infiltration pattern : simulink/Signal Routing/Manual Switch  SystemSampleTime=-1  sw=1  action=0  varsize=off
  Out1 : Outport  OutDataType=sfix(16)  OutScaling=2^0
  wires:
  switch ON/OFF  infiltration pattern/1 -> Sum/1
  Sum/1 -> Saturation/1
  Saturation/1 -> Gain1/1
  Gain1/1 -> Out1/1, To Workspace1/1
  Random Number  IndS Flow rate/1 -> Sum/2
  Sine Wave/1 -> switch ON/OFF  infiltration pattern/1
  Constant/1 -> switch ON/OFF  infiltration pattern/2

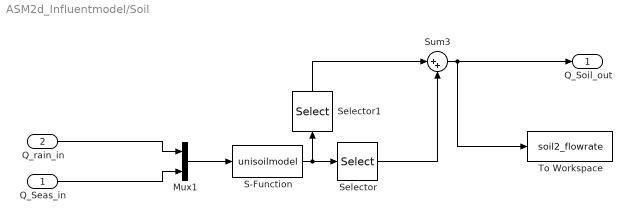
== system ASM2d_Influentmodel/Soil ==
  Q_Seas_in : Inport  OutDataType=sfix(16)  OutScaling=2^0
  Q_rain_in : Inport  Port=2  OutDataType=sfix(16)  OutScaling=2^0
  Mux1 : Mux  Inputs=2
  S-Function : S-Function  FunctionName=unisoilmodel  Parameters=XINITSOIL, PARS_SOIL
  Selector : Selector  InputPortWidth=4  IndexOptions=Index vector (dialog)  Indices=[1]  OutputSizes=1
  Selector1 : Selector  Orientation=up  InputPortWidth=4  IndexOptions=Index vector (dialog)  Indices=[2]  OutputSizes=1
  Sum3 : Sum  Inputs=|++  OutDataType=sfix(16)  OutScaling=2^0  SaturateOnIntegerOverflow=on
  To Workspace : ToWorkspace  VariableName=soil2_flowrate  SampleTime=-1  SaveFormat=Array
  Q_Soil_out : Outport
  wires:
  S-Function/1 -> Selector/1, Selector1/1
  Selector1/1 -> Sum3/1
  Selector/1 -> Sum3/2
  Sum3/1 -> Q_Soil_out/1, To Workspace/1
  Mux1/1 -> S-Function/1
  Q_rain_in/1 -> Mux1/1
  Q_Seas_in/1 -> Mux1/2

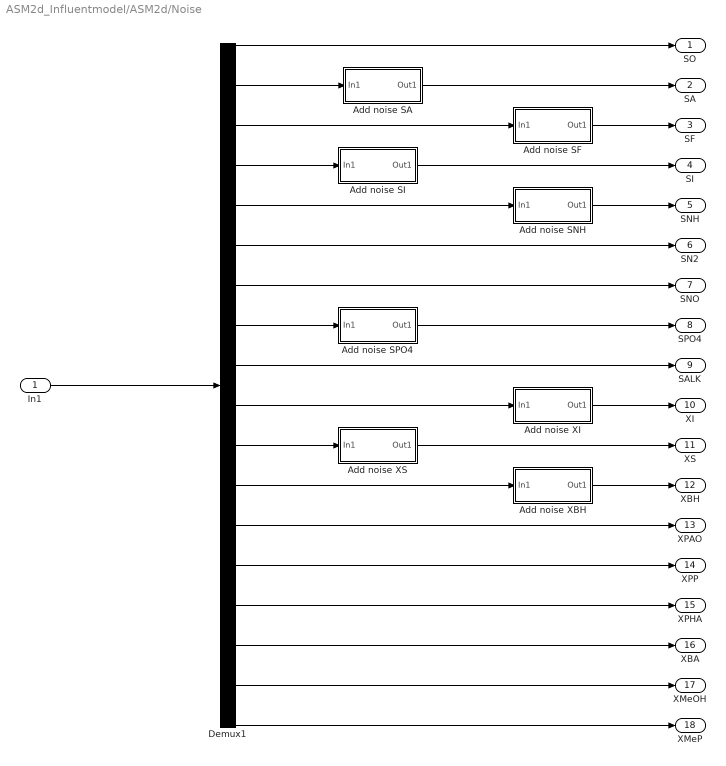
== system ASM2d_Influentmodel/ASM2d/Noise ==
  In1 : Inport  OutDataType=sfix(16)  OutScaling=2^0
  Add noise SA : Subsystem
  Add noise SF : Subsystem
  Add noise SI : Subsystem
  Add noise SNH : Subsystem
  Add noise SPO4 : Subsystem
  Add noise XBH : Subsystem
  Add noise XI : Subsystem
  Add noise XS : Subsystem
  Demux1 : Demux  Outputs=[1 1 1 1 1 1 1 1 1 1 1 1 1 1 1 1 1 1]
  SO : Outport  OutDataType=sfix(16)  OutScaling=2^0
  SA : Outport  Port=2  OutDataType=sfix(16)  OutScaling=2^0
  SF : Outport  Port=3  OutDataType=sfix(16)  OutScaling=2^0
  SI : Outport  Port=4  OutDataType=sfix(16)  OutScaling=2^0
  SNH : Outport  Port=5  OutDataType=sfix(16)  OutScaling=2^0
  SN2 : Outport  Port=6  OutDataType=sfix(16)  OutScaling=2^0
  SNO : Outport  Port=7  OutDataType=sfix(16)  OutScaling=2^0
  SPO4 : Outport  Port=8  OutDataType=sfix(16)  OutScaling=2^0
  SALK : Outport  Port=9  OutDataType=sfix(16)  OutScaling=2^0
  XI : Outport  Port=10  OutDataType=sfix(16)  OutScaling=2^0
  XS : Outport  Port=11  OutDataType=sfix(16)  OutScaling=2^0
  XBH : Outport  Port=12  OutDataType=sfix(16)  OutScaling=2^0
  XPAO : Outport  Port=13  OutDataType=sfix(16)  OutScaling=2^0
  XPP : Outport  Port=14  OutDataType=sfix(16)  OutScaling=2^0
  XPHA : Outport  Port=15  OutDataType=sfix(16)  OutScaling=2^0
  XBA : Outport  Port=16  OutDataType=sfix(16)  OutScaling=2^0
  XMeOH : Outport  Port=17  OutDataType=sfix(16)  OutScaling=2^0
  XMeP : Outport  Port=18  OutDataType=sfix(16)  OutScaling=2^0
  wires:
  Add noise SA/1(Out1) -> SA/1
  Demux1/2 -> Add noise SA/1(In1)
  Add noise SF/1(Out1) -> SF/1
  Demux1/3 -> Add noise SF/1(In1)
  Demux1/4 -> Add noise SI/1(In1)
  Add noise SI/1(Out1) -> SI/1
  Demux1/5 -> Add noise SNH/1(In1)
  Add noise SNH/1(Out1) -> SNH/1
  Demux1/7 -> SNO/1
  Demux1/8 -> Add noise SPO4/1(In1)
  Add noise SPO4/1(Out1) -> SPO4/1
  Demux1/9 -> SALK/1
  Add noise XI/1(Out1) -> XI/1
  Demux1/10 -> Add noise XI/1(In1)
  Add noise XS/1(Out1) -> XS/1
  Demux1/11 -> Add noise XS/1(In1)
  Demux1/12 -> Add noise XBH/1(In1)
  Add noise XBH/1(Out1) -> XBH/1
  Demux1/16 -> XBA/1
  Demux1/13 -> XPAO/1
  Demux1/14 -> XPP/1
  Demux1/15 -> XPHA/1
  Demux1/17 -> XMeOH/1
  In1/1 -> Demux1/1
  Demux1/6 -> SN2/1
  Demux1/18 -> XMeP/1
  Demux1/1 -> SO/1

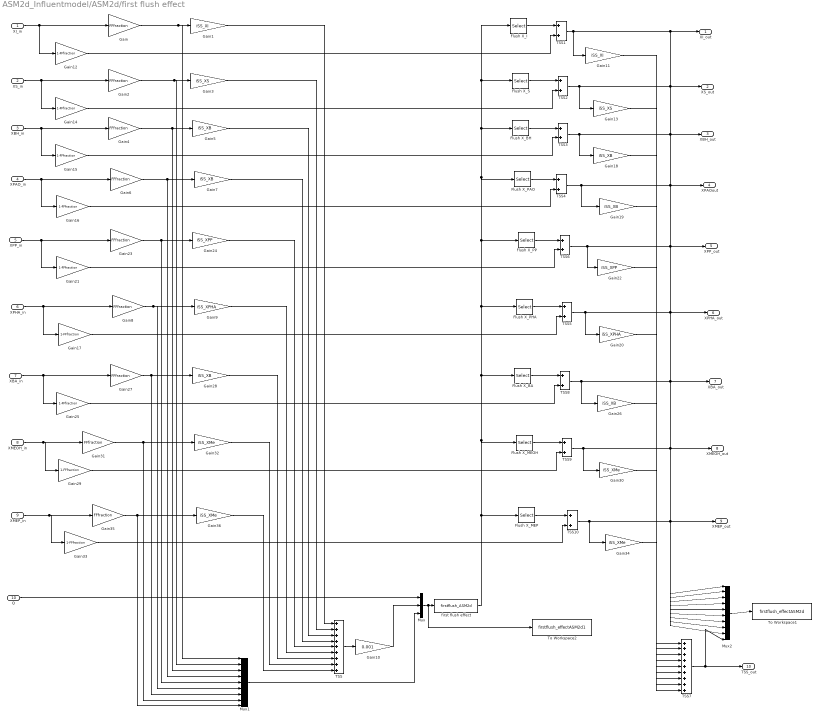
== system ASM2d_Influentmodel/ASM2d/first flush effect ==
  XI_in : Inport  OutDataType=sfix(16)  OutScaling=2^0
  XS_in : Inport  Port=2  OutDataType=sfix(16)  OutScaling=2^0
  XBH_in : Inport  Port=3  OutDataType=sfix(16)  OutScaling=2^0
  XPAO_in : Inport  Port=4  OutDataType=sfix(16)  OutScaling=2^0
  XPP_in : Inport  Port=5  OutDataType=sfix(16)  OutScaling=2^0
  XPHA_in : Inport  Port=6  OutDataType=sfix(16)  OutScaling=2^0
  XBA_in : Inport  Port=7  OutDataType=sfix(16)  OutScaling=2^0
  XMEOH_in : Inport  Port=8  OutDataType=sfix(16)  OutScaling=2^0
  XMEP_in : Inport  Port=9  OutDataType=sfix(16)  OutScaling=2^0
  Q : Inport  Port=10  OutDataType=sfix(16)  OutScaling=2^0
  Flush X_BA : Selector  InputPortWidth=21  IndexOptions=Index vector (dialog)  Indices=[9]  OutputSizes=1
  Flush X_BH : Selector  InputPortWidth=21  IndexOptions=Index vector (dialog)  Indices=[5]  OutputSizes=1
  Flush X_I : Selector  InputPortWidth=21  IndexOptions=Index vector (dialog)  Indices=[3]  OutputSizes=1
  Flush X_MEOH : Selector  InputPortWidth=21  IndexOptions=Index vector (dialog)  Indices=[10]  OutputSizes=1
  Flush X_MEP : Selector  InputPortWidth=21  IndexOptions=Index vector (dialog)  Indices=[11]  OutputSizes=1
  Flush X_PAO : Selector  InputPortWidth=21  IndexOptions=Index vector (dialog)  Indices=[6]  OutputSizes=1
  Flush X_PHA : Selector  InputPortWidth=21  IndexOptions=Index vector (dialog)  Indices=[8]  OutputSizes=1
  Flush X_PP : Selector  InputPortWidth=21  IndexOptions=Index vector (dialog)  Indices=[7]  OutputSizes=1
  Flush X_S : Selector  InputPortWidth=21  IndexOptions=Index vector (dialog)  Indices=[4]  OutputSizes=1
  Gain{,2,4,6,8,23,27,31,35} (9 alike) : Gain  Gain=FFfraction  ParameterDataType=sfix(16)  ParameterScaling=2^0  OutDataType=sfix(16)  OutScaling=2^0
  Gain1 : Gain  Gain=iSS_XI  ParameterDataType=sfix(16)  ParameterScaling=2^0  OutDataType=sfix(16)  OutScaling=2^0
  Gain10 : Gain  Gain=0.001  ParameterDataType=sfix(16)  ParameterScaling=2^0  OutDataType=sfix(16)  OutScaling=2^0
  Gain11 : Gain  Gain=iSS_XI  ParameterDataType=sfix(16)  ParameterScaling=2^0  OutDataType=sfix(16)  OutScaling=2^0
  Gain{12,14..17,21,25,29,33} (9 alike) : Gain  Gain=1-FFfraction  ParameterDataType=sfix(16)  ParameterScaling=2^0  OutDataType=sfix(16)  OutScaling=2^0
  Gain13 : Gain  Gain=iSS_XS  ParameterDataType=sfix(16)  ParameterScaling=2^0  OutDataType=sfix(16)  OutScaling=2^0
  Gain{5,7,18..19,26,28} (6 alike) : Gain  Gain=iSS_XB  ParameterDataType=sfix(16)  ParameterScaling=2^0  OutDataType=sfix(16)  OutScaling=2^0
  Gain20 : Gain  Gain=iSS_XPHA  ParameterDataType=sfix(16)  ParameterScaling=2^0  OutDataType=sfix(16)  OutScaling=2^0
  Gain22 : Gain  Gain=iSS_XPP  ParameterDataType=sfix(16)  ParameterScaling=2^0  OutDataType=sfix(16)  OutScaling=2^0
  Gain24 : Gain  Gain=iSS_XPP  ParameterDataType=sfix(16)  ParameterScaling=2^0  OutDataType=sfix(16)  OutScaling=2^0
  Gain3 : Gain  Gain=iSS_XS  ParameterDataType=sfix(16)  ParameterScaling=2^0  OutDataType=sfix(16)  OutScaling=2^0
  Gain{30,32,34,36} (4 alike) : Gain  Gain=iSS_XMe  ParameterDataType=sfix(16)  ParameterScaling=2^0  OutDataType=sfix(16)  OutScaling=2^0
  Gain9 : Gain  Gain=iSS_XPHA  ParameterDataType=sfix(16)  ParameterScaling=2^0  OutDataType=sfix(16)  OutScaling=2^0
  Mux : Mux  Inputs=3
  Mux1 : Mux  Inputs=9
  Mux2 : Mux  Inputs=10
  TSS : Sum  Inputs=+++++++++  OutDataType=sfix(16)  OutScaling=2^-10
  TSS{1..6,8..10} (9 alike) : Sum  OutDataType=sfix(16)  OutScaling=2^-10
  TSS7 : Sum  Inputs=+++++++++  OutDataType=sfix(16)  OutScaling=2^-10
  To Workspace1 : ToWorkspace  VariableName=firstflush_effectASM2d  SampleTime=-1  SaveFormat=Array
  To Workspace2 : ToWorkspace  VariableName=firstflush_effectASM2d1  SampleTime=-1  SaveFormat=Array
  first flush effect : S-Function  FunctionName=firstflush_ASM2d  Parameters=ASM2d_XINIT, SSPARS
  XI_out : Outport  OutDataType=sfix(16)  OutScaling=2^0
  XS_out : Outport  Port=2  OutDataType=sfix(16)  OutScaling=2^0
  XBH_out : Outport  Port=3  OutDataType=sfix(16)  OutScaling=2^0
  XPAOout : Outport  Port=4  OutDataType=sfix(16)  OutScaling=2^0
  XPP_out : Outport  Port=5  OutDataType=sfix(16)  OutScaling=2^0
  XPHA_out : Outport  Port=6  OutDataType=sfix(16)  OutScaling=2^0
  XBA_out : Outport  Port=7  OutDataType=sfix(16)  OutScaling=2^0
  XMEOH_out : Outport  Port=8  OutDataType=sfix(16)  OutScaling=2^0
  XMEP_out : Outport  Port=9  OutDataType=sfix(16)  OutScaling=2^0
  TSS_out : Outport  Port=10  OutDataType=sfix(16)  OutScaling=2^0
  wires:
  XI_in/1 -> Gain/1, Gain12/1
  Gain/1 -> Gain1/1, Mux1/1
  XS_in/1 -> Gain2/1, Gain14/1
  Gain2/1 -> Gain3/1, Mux1/2
  XBH_in/1 -> Gain4/1, Gain15/1
  Gain4/1 -> Gain5/1, Mux1/3
  XPAO_in/1 -> Gain6/1, Gain16/1
  Gain6/1 -> Gain7/1, Mux1/4
  Mux1/1 -> Mux/3
  Q/1 -> Mux/1
  Mux/1 -> first flush effect/1, To Workspace2/1
  TSS/1 -> Gain10/1
  Gain10/1 -> Mux/2
  Gain12/1 -> TSS1/2
  Flush X_I/1 -> TSS1/1
  Flush X_S/1 -> TSS2/1
  Gain14/1 -> TSS2/2
  Flush X_BH/1 -> TSS3/1
  Gain15/1 -> TSS3/2
  Gain16/1 -> TSS4/2
  Flush X_PAO/1 -> TSS4/1
  TSS3/1 -> Gain18/1, XBH_out/1, Mux2/3
  Mux2/1 -> To Workspace1/1
  XMEOH_in/1 -> Gain29/1, Gain31/1
  Flush X_MEOH/1 -> TSS9/1
  TSS9/1 -> Gain30/1, XMEOH_out/1
  Gain31/1 -> Gain32/1, Mux1/8
  Gain33/1 -> TSS10/2
  XMEP_in/1 -> Gain33/1, Gain35/1
  Flush X_MEP/1 -> TSS10/1
  TSS10/1 -> Gain34/1, XMEP_out/1
  Gain35/1 -> Gain36/1, Mux1/9
  XPP_in/1 -> Gain21/1, Gain23/1
  Gain21/1 -> TSS6/2
  Gain23/1 -> Gain24/1, Mux1/5
  Flush X_PP/1 -> TSS6/1
  TSS6/1 -> Gain22/1, XPP_out/1, Mux2/5
  Gain27/1 -> Gain28/1, Mux1/7
  Gain25/1 -> TSS8/2
  XBA_in/1 -> Gain27/1, Gain25/1
  Flush X_BA/1 -> TSS8/1
  TSS8/1 -> Gain26/1, XBA_out/1, Mux2/7
  XPHA_in/1 -> Gain8/1, Gain17/1
  Gain8/1 -> Gain9/1, Mux1/6
  Gain17/1 -> TSS5/2
  Flush X_PHA/1 -> TSS5/1
  TSS2/1 -> Gain13/1, XS_out/1, Mux2/2
  TSS1/1 -> Gain11/1, XI_out/1, Mux2/1
  TSS4/1 -> Gain19/1, XPAOout/1, Mux2/4
  TSS5/1 -> Gain20/1, XPHA_out/1, Mux2/6, Mux2/8, Mux2/9
  Gain29/1 -> TSS9/2
  Gain1/1 -> TSS/1
  Gain3/1 -> TSS/2
  Gain5/1 -> TSS/3
  Gain7/1 -> TSS/4
  Gain24/1 -> TSS/5
  Gain9/1 -> TSS/6
  Gain28/1 -> TSS/7
  Gain32/1 -> TSS/8
  Gain36/1 -> TSS/9
  first flush effect/1 -> Flush X_I/1, Flush X_S/1, Flush X_BH/1, Flush X_PAO/1, Flush X_PP/1, Flush X_PHA/1, Flush X_BA/1, Flush X_MEOH/1, Flush X_MEP/1
  Gain11/1 -> TSS7/1
  Gain13/1 -> TSS7/2
  Gain18/1 -> TSS7/3
  Gain19/1 -> TSS7/4
  Gain22/1 -> TSS7/5
  Gain20/1 -> TSS7/6
  Gain26/1 -> TSS7/7
  Gain30/1 -> TSS7/8
  Gain34/1 -> TSS7/9
  TSS7/1 -> Mux2/10, TSS_out/1

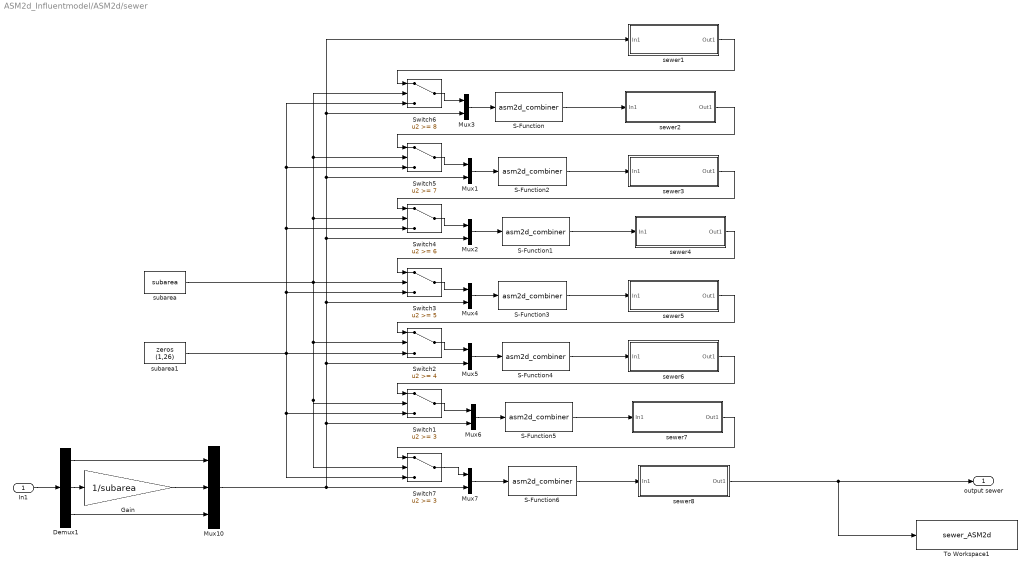
== system ASM2d_Influentmodel/ASM2d/sewer ==
  In1 : Inport  OutDataType=sfix(16)  OutScaling=2^0
  Demux1 : Demux  Outputs=[19 1 6]
  Gain : Gain  Gain=1/subarea  ParameterDataType=sfix(16)  ParameterScaling=2^0  OutDataType=sfix(16)  OutScaling=2^0
  Mux{1..7} (7 alike) : Mux  Inputs=2
  Mux10 : Mux  Inputs=3
  S-Function{,1..6} (7 alike) : S-Function  FunctionName=asm2d_combiner
  Switch1 : Switch  Threshold=3  SaturateOnIntegerOverflow=on
  Switch2 : Switch  Threshold=4  SaturateOnIntegerOverflow=on
  Switch3 : Switch  Threshold=5  SaturateOnIntegerOverflow=on
  Switch4 : Switch  Threshold=6  SaturateOnIntegerOverflow=on
  Switch5 : Switch  Threshold=7  SaturateOnIntegerOverflow=on
  Switch6 : Switch  Threshold=8  SaturateOnIntegerOverflow=on
  Switch7 : Switch  Threshold=3  SaturateOnIntegerOverflow=on
  To Workspace1 : ToWorkspace  VariableName=sewer_ASM2d  SampleTime=-1  SaveFormat=Array
  sewer1 : Subsystem
  sewer2 : Subsystem
  sewer3 : Subsystem
  sewer4 : Subsystem
  sewer5 : Subsystem
  sewer6 : Subsystem
  sewer7 : Subsystem
  sewer8 : Subsystem
  subarea : Constant  Value=subarea  OutDataType=sfix(16)  OutScaling=2^0
  subarea1 : Constant  Value=zeros (1,26)  OutDataType=sfix(16)  OutScaling=2^0
  output sewer : Outport  OutDataType=sfix(16)  OutScaling=2^0
  wires:
  In1/1 -> Demux1/1
  Demux1/2 -> Gain/1
  Demux1/1 -> Mux10/1
  Demux1/3 -> Mux10/3
  Gain/1 -> Mux10/2
  S-Function/1 -> sewer2/1(In1)
  sewer2/1(Out1) -> Switch5/1
  S-Function2/1 -> sewer3/1(In1)
  sewer3/1(Out1) -> Switch4/1
  S-Function1/1 -> sewer4/1(In1)
  sewer4/1(Out1) -> Switch3/1
  S-Function3/1 -> sewer5/1(In1)
  sewer5/1(Out1) -> Switch2/1
  sewer1/1(Out1) -> Switch6/1
  S-Function4/1 -> sewer6/1(In1)
  sewer6/1(Out1) -> Switch1/1
  S-Function5/1 -> sewer7/1(In1)
  sewer7/1(Out1) -> Switch7/1
  S-Function6/1 -> sewer8/1(In1)
  Mux10/1 -> Mux1/2, Mux3/2, sewer1/1(In1), Mux2/2, Mux4/2, Mux5/2, Mux6/2, Mux7/2
  Switch6/1 -> Mux3/1
  Mux3/1 -> S-Function/1
  Switch5/1 -> Mux1/1
  Switch4/1 -> Mux2/1
  Switch3/1 -> Mux4/1
  Switch1/1 -> Mux6/1
  Switch2/1 -> Mux5/1
  Switch7/1 -> Mux7/1
  Mux1/1 -> S-Function2/1
  Mux2/1 -> S-Function1/1
  Mux4/1 -> S-Function3/1
  Mux5/1 -> S-Function4/1
  Mux6/1 -> S-Function5/1
  Mux7/1 -> S-Function6/1
  sewer8/1(Out1) -> output sewer/1, To Workspace1/1
  subarea/1 -> Switch3/2, Switch6/2, Switch5/2, Switch4/2, Switch2/2, Switch7/2, Switch1/2
  subarea1/1 -> Switch2/3, Switch6/3, Switch5/3, Switch4/3, Switch3/3, Switch1/3, Switch7/3

== system ASM2d_Influentmodel/ASM2d/Noise/Add noise SA ==
  In1 : Inport  OutDataType=sfix(16)  OutScaling=2^0
  Random Number : RandomNumber  Variance=SA_nv*polnoiseswitch  Seed=SA_ns  SampleTime=SA_st
  Saturation : Saturate  UpperLimit=SA_max  LowerLimit=SA_min
  Sum : Sum  Inputs=|++  OutDataType=sfix(16)  OutScaling=2^0  SaturateOnIntegerOverflow=on
  Out1 : Outport
  wires:
  Sum/1 -> Saturation/1
  Random Number/1 -> Sum/2
  Saturation/1 -> Out1/1
  In1/1 -> Sum/1

== system ASM2d_Influentmodel/ASM2d/Noise/Add noise SF ==
  In1 : Inport  OutDataType=sfix(16)  OutScaling=2^0
  Random Number : RandomNumber  Variance=SF_nv*polnoiseswitch  Seed=SF_ns  SampleTime=SF_st
  Saturation : Saturate  UpperLimit=SF_max  LowerLimit=SF_min
  Sum : Sum  Inputs=|++  OutDataType=sfix(16)  OutScaling=2^0  SaturateOnIntegerOverflow=on
  Out1 : Outport
  wires:
  Sum/1 -> Saturation/1
  Random Number/1 -> Sum/2
  Saturation/1 -> Out1/1
  In1/1 -> Sum/1

== system ASM2d_Influentmodel/ASM2d/Noise/Add noise SI ==
  In1 : Inport  OutDataType=sfix(16)  OutScaling=2^0
  Random Number : RandomNumber  Variance=SI_nv*polnoiseswitch  Seed=SI_ns  SampleTime=SI_st
  Saturation : Saturate  UpperLimit=SI_max  LowerLimit=SI_min
  Sum : Sum  Inputs=|++  OutDataType=sfix(16)  OutScaling=2^0  SaturateOnIntegerOverflow=on
  Out1 : Outport
  wires:
  Sum/1 -> Saturation/1
  Random Number/1 -> Sum/2
  Saturation/1 -> Out1/1
  In1/1 -> Sum/1

== system ASM2d_Influentmodel/ASM2d/Noise/Add noise SNH ==
  In1 : Inport  OutDataType=sfix(16)  OutScaling=2^0
  Random Number : RandomNumber  Variance=SNH_nv*polnoiseswitch  Seed=SNH_ns  SampleTime=SNH_st
  Saturation : Saturate  UpperLimit=SNH_max  LowerLimit=SNH_min
  Sum : Sum  Inputs=|++  OutDataType=sfix(16)  OutScaling=2^0  SaturateOnIntegerOverflow=on
  Out1 : Outport
  wires:
  Sum/1 -> Saturation/1
  Random Number/1 -> Sum/2
  Saturation/1 -> Out1/1
  In1/1 -> Sum/1

== system ASM2d_Influentmodel/ASM2d/Noise/Add noise SPO4 ==
  In1 : Inport  OutDataType=sfix(16)  OutScaling=2^0
  Random Number : RandomNumber  Variance=SPO4_nv*polnoiseswitch  Seed=SPO4_ns  SampleTime=SPO4_st
  Saturation : Saturate  UpperLimit=SNH_max  LowerLimit=SNH_min
  Sum : Sum  Inputs=|++  OutDataType=sfix(16)  OutScaling=2^0  SaturateOnIntegerOverflow=on
  Out1 : Outport
  wires:
  Sum/1 -> Saturation/1
  Random Number/1 -> Sum/2
  Saturation/1 -> Out1/1
  In1/1 -> Sum/1

== system ASM2d_Influentmodel/ASM2d/Noise/Add noise XBH ==
  In1 : Inport  OutDataType=sfix(16)  OutScaling=2^0
  Random Number : RandomNumber  Variance=XBH_nv*polnoiseswitch  Seed=XBH_ns  SampleTime=XBH_st
  Saturation : Saturate  UpperLimit=XBH_max  LowerLimit=XBH_min
  Sum : Sum  Inputs=|++  OutDataType=sfix(16)  OutScaling=2^0  SaturateOnIntegerOverflow=on
  Out1 : Outport
  wires:
  Sum/1 -> Saturation/1
  Random Number/1 -> Sum/2
  Saturation/1 -> Out1/1
  In1/1 -> Sum/1

== system ASM2d_Influentmodel/ASM2d/Noise/Add noise XI ==
  In1 : Inport  OutDataType=sfix(16)  OutScaling=2^0
  Random Number : RandomNumber  Variance=XI_nv*polnoiseswitch  Seed=XI_ns  SampleTime=XI_st
  Saturation : Saturate  UpperLimit=XI_max  LowerLimit=XI_min
  Sum : Sum  Inputs=|++  OutDataType=sfix(16)  OutScaling=2^0  SaturateOnIntegerOverflow=on
  Out1 : Outport
  wires:
  Sum/1 -> Saturation/1
  Random Number/1 -> Sum/2
  Saturation/1 -> Out1/1
  In1/1 -> Sum/1

== system ASM2d_Influentmodel/ASM2d/Noise/Add noise XS ==
  In1 : Inport  OutDataType=sfix(16)  OutScaling=2^0
  Random Number : RandomNumber  Variance=XS_nv*polnoiseswitch  Seed=XS_ns  SampleTime=XS_st
  Saturation : Saturate  UpperLimit=XS_max  LowerLimit=XS_min
  Sum : Sum  Inputs=|++  OutDataType=sfix(16)  OutScaling=2^0  SaturateOnIntegerOverflow=on
  Out1 : Outport
  wires:
  Sum/1 -> Saturation/1
  Random Number/1 -> Sum/2
  Saturation/1 -> Out1/1
  In1/1 -> Sum/1

== system ASM2d_Influentmodel/ASM2d/sewer/sewer1 ==
  In1 : Inport  OutDataType=sfix(16)  OutScaling=2^0
  Constant : Constant  OutDataType=sfix(16)  OutScaling=2^0
  Mux1 : Mux  Inputs=2
  S-Function : S-Function  FunctionName=sewer_asm2d  Parameters=ASM2d_SEWERINIT, ASM2d_PARS, SPAR
  S-Function1 : S-Function  FunctionName=sewer_asm2d  Parameters=ASM2d_SEWERINIT, ASM2d_PARS, SPAR
  S-Function2 : S-Function  FunctionName=sewer_asm2d  Parameters=ASM2d_SEWERINIT, ASM2d_PARS, SPAR
  Selector9 : Selector  InputPortWidth=27  IndexOptions=Index vector (dialog)  Indices=[1 2 3 4 5 6 7 8 9 10 11 12 13 14 15 16 17 18 19 20 21 22 23 24 25 26 ]  OutputSizes=1
  Out1 : Outport
  wires:
  S-Function/1 -> S-Function1/1
  S-Function1/1 -> S-Function2/1
  S-Function2/1 -> Selector9/1
  Mux1/1 -> S-Function/1
  Constant/1 -> Mux1/2
  In1/1 -> Mux1/1
  Selector9/1 -> Out1/1

== system ASM2d_Influentmodel/ASM2d/sewer/sewer2 ==
  In1 : Inport  OutDataType=sfix(16)  OutScaling=2^0
  Constant : Constant  OutDataType=sfix(16)  OutScaling=2^0
  Mux1 : Mux  Inputs=2
  S-Function : S-Function  FunctionName=sewer_asm2d  Parameters=ASM2d_SEWERINIT, ASM2d_PARS, SPAR
  S-Function1 : S-Function  FunctionName=sewer_asm2d  Parameters=ASM2d_SEWERINIT, ASM2d_PARS, SPAR
  S-Function2 : S-Function  FunctionName=sewer_asm2d  Parameters=ASM2d_SEWERINIT, ASM2d_PARS, SPAR
  Selector9 : Selector  InputPortWidth=27  IndexOptions=Index vector (dialog)  Indices=[1 2 3 4 5 6 7 8 9 10 11 12 13 14 15 16 17 18 19 20 21 22 23 24 25 26 ]  OutputSizes=1
  Out1 : Outport
  wires:
  S-Function/1 -> S-Function1/1
  S-Function1/1 -> S-Function2/1
  S-Function2/1 -> Selector9/1
  Mux1/1 -> S-Function/1
  Constant/1 -> Mux1/2
  In1/1 -> Mux1/1
  Selector9/1 -> Out1/1

== system ASM2d_Influentmodel/ASM2d/sewer/sewer3 ==
  In1 : Inport  OutDataType=sfix(16)  OutScaling=2^0
  Constant : Constant  OutDataType=sfix(16)  OutScaling=2^0
  Mux1 : Mux  Inputs=2
  S-Function : S-Function  FunctionName=sewer_asm2d  Parameters=ASM2d_SEWERINIT, ASM2d_PARS, SPAR
  S-Function1 : S-Function  FunctionName=sewer_asm2d  Parameters=ASM2d_SEWERINIT, ASM2d_PARS, SPAR
  S-Function2 : S-Function  FunctionName=sewer_asm2d  Parameters=ASM2d_SEWERINIT, ASM2d_PARS, SPAR
  Selector9 : Selector  InputPortWidth=27  IndexOptions=Index vector (dialog)  Indices=[1 2 3 4 5 6 7 8 9 10 11 12 13 14 15 16 17 18 19 20 21 22 23 24 25 26 ]  OutputSizes=1
  Out1 : Outport
  wires:
  S-Function/1 -> S-Function1/1
  S-Function1/1 -> S-Function2/1
  S-Function2/1 -> Selector9/1
  Mux1/1 -> S-Function/1
  Constant/1 -> Mux1/2
  In1/1 -> Mux1/1
  Selector9/1 -> Out1/1
